simulink model "self_triggered_mpc_simulation"  (R2023a)
settings: Solver=VariableStepAuto  StartTime=0.0  StopTime=1  RelTol=1e-3
values from neighbouring files (symbols this model uses):
  param = param_setup()    [cost_cal.m]    (also in main.m; param.mat = ; self_triggered_mpc_heemels.m)
(part 2 of 2)

== stateflow chart self_triggered_mpc_simulation/Chart ==
  state self_triggered_mpc_autometica_ver
    state triggering_confirm
    state implement_mpc
      entry:
      [nTM,input]=autometica_mpc(rtm, state)
      control = input;
      during:
      [nTM,input]=autometica_mpc(rtm, state)
      control = input;
    state holding
      entry:
      control = input;
      nTM = 0;
      %holding시 nTM은 안쓰므로
      %쓰래기값을 주어도 됨
      during:
      control = input;
      nTM = 0;
    (default) -> triggering_confirm
    triggering_confirm -> implement_mpc [order 1] : [triggering == 1]
    triggering_confirm -> holding [order 2] : [triggering == 0]
    holding -> implement_mpc : [triggering == 1]
    implement_mpc -> holding : [triggering == 0]
  (default) -> self_triggered_mpc_autometica_ver
  data: TM function_input; state function_input; nTM function_output; input function_output; tm function_input; tmarr function_output; marker function_output; tm function_input; tmarr function_output; marker function_output; tm function_input; tmarr function_output; marker function_output; tm function_input; tmarr function_output; marker function_output; tm function_input; tmarr function_output; marker function_output; tm function_input; tmarr function_output; marker function_output; tm function_input; tmarr function_output; marker function_output; tm function_input; tmarr function_output; marker function_output; tm function_input; tmarr function_output; marker function_output; trigger input; rtm input; state input; nTM output; control output; input local
  function [nTM, input] = autometica_mpc(TM, state):
    | function [nTM, input] = autometica_mpc(TM, state)
    | 
    |     coder.extrinsic("optimconstr", "optimproblem", "optimvar");
    | %==========================================================================
    |  %parameter setting
    |     param = load("param.mat");
    |     param = param.param;
    |     Nl = size(TM);
    |     param.N = Nl(2);
    | %==========================================================================
    |     %implement autometica vesion
    |     prob = optimproblem;
    |     x0 = optimvar('x0', param.nx);
    |     x = optimvar('x', param.nx, param.N);
    |     u0 = optimvar('u0', param.nu);
    |     u = optimvar('u',param.nu, (param.N)-1);
    |     size(u)
    |     cost_function =x0'*param.Q*x0+u0*param.R*u0;
    |     for i=1:param.N-1
    |         cost_function = cost_function + x(:,i)'*param.Q*x(:,i) + u(:,i)'*param.R*u(:,i); % terminal cost 설정해야 됨
    |     end
    |     prob.Objective = cost_function;
    |     
    | %==========================================================================
    | % model constraints
    | 
    |     model_constr = optimconstr(param.nx,(param.N)+1);
    |     model_constr(:,1) = x(:,1) == param.A*x0 + param.B*u0;
    |     for i=1:param.N-1
    |         model_constr(:,i+1) = x(:,i+1) == param.A*x(:,i) + param.B*u(:,i);
    |     end
    |     model_constr(:,(param.N)+1) = x0 == state;
    |     prob.Constraints.model_constr = model_constr;
    |     
    | %==========================================================================
    | %terminal set constraints
    |     constT = optimconstr(30,param.autometica_Tset+1);
    |        
    |     LL = param.tildeF - param.tildeG*param.tildeK;
    |     for i= 1:param.autometica_Tset
    |         constT(:,i) = LL*(param.A_BK^(i))*param.phi(:,1:2)*x(:,param.N)<=ones(30,1);
    |     end
    |     constT(1:param.NumOfConstr,param.autometica_Tset+1) = (param.F-param.G*param.K)*x(:,param.N)<=1;
    |     prob.Constraints.ConstT = constT;
    | %==========================================================================
    | % triggering constraints
    |     SizeOfTM = size(TM);
    |     tm = TM(2:SizeOfTM(2));
    |     SizeOftm = size(tm);
    |     tmcomp = find(tm);
    |     SizeOfTmcomp = size(tmcomp);
    |     % triggering_constr = optimconstr(param.N);
    |     % triggering_constr(1) = u0 == u(:,1);
    |     % for i = 1:param.N-2
    |     %     triggering_constr(i+1) = u(:,i)==u(:,i+1); %% i+1에서 triggering하면 u(:,i)~=u(:,i+1)
    |     % end
    |     % for i = 1:SizeOfTmcomp %% required triggering time moment setting
    |     %     if tmcomp(i)==1
    |     %         triggering_constr(tmcopm(i)) = u0 ~= u(:,1);
    |     %     else
    |     %         triggering_constr(tmcomp(i)) =  u(:,tmcomp(i)-1) ~= u(:,tmcomp(i));
    |     %     end
    |     % end
    |     nontm = find(~tm); 
    |     SizeOfnontm = size(nontm);
    | %==========================================================================
    | % required trigger time moment sequence에서 triggering time moment 추가하기
    | % 이부분에서 tmarr marker를 결과로 얻는데 tmarr는 triggering time moment sequence에서
    | % triggering time moment를 추가하여 얻을 수 있는 모든 sequence를 묶어 tmarr로 받는다
    | 
    |     tmarr = [];
    |     switch SizeOfnontm(2)
    |         case 9
    |             [tmarr, marker] = trigger_plus_9(tm);
    |         case 8
    |             [tmarr, marker] = trigger_plus_8(tm);
    |         case 7
    |             [tmarr, marker] = trigger_plus_7(tm);
    |         case 6
    |             [tmarr, marker] = trigger_plus_6(tm);
    |         case 5
    |             [tmarr, marker] = trigger_plus_5(tm);
    |         case 4
    |             [tmarr, marker] = trigger_plus_4(tm);
    |         case 3
    |             [tmarr, marker] = trigger_plus_3(tm);
    |         case 2
    |             [tmarr, marker] = trigger_plus_2(tm);
    |         case 1
    |             [tmarr, marker] = trigger_plus_1(tm);
    |         case 0
    |             [tmarr, marker] = trigger_plus_0(tm);
    |     end
    | 
    | %==========================================================================
    | 
    |     SizeOftmarr = size(tmarr);
    |     SizeOfmarker = size(marker);
    | 
    |     % triggering_constr = optimconstr(param.nu, SizeOftm(2));
    |     % triggering_constr(:,1) = u0 == u(:,1); %SizeOfTM == param.N
    |     % for i = 2:SizeOftm(2)
    |     %     triggering_constr(:,i) = u(:,i-1)==u(:,i); %% i+1에서 triggering하면 u(:,i)~=u(:,i+1)
    |     % end
    |     solArr = [];
    |     fvalArr = [];
    |     exitflagArr = [];
    |     for i = 1:SizeOfmarker(2)
    |         for j = marker(i):marker(i+1)-1 
    | 
    |             tm_setting = tmarr(j,:)
    |             triggering_constr = optimconstr(param.nu, SizeOftm(2));%tm이 정해짐
    | 
    |             for k = 1:SizeOftm(2) %% required triggering time moment setting
    |                 k
    |                 if  tm_setting(k) == 0
    |                     if k ==1
    |                         triggering_constr(:,k) = u0 == u(:,1) %%optimconstr에서 ~=가 지원되지 않음
    |                         show(triggering_constr(:,k))
    |                     else
    |                         size(triggering_constr(:,k))
    |                         size(u)
    |                         triggering_constr(:,k) =  u(:,k-1) == u(:,k)
    |                         show(triggering_constr(:,i))
    |                     end
    |                 end
    |             end
    |             prob.Constraints.triggering_constr = triggering_constr
    |             [sol,fval,exitflag,output,lambda] = solve(prob)
    |             solArr = [solArr sol]
    |             fvalArr = [fvalArr fval]
    |             exitflagArr = [exitflagArr exitflag]
    |         end
    | 
    |         if ~isempty(exitflagArr==1)
    |             temp = min(fvalArr);
    |             [row, col] = find(fvalArr == temp);
    |             input=solArr(row, col).u0;
    |             nTM = tmarr(marker(i)+col-1,:);
    |             return;
    |         end
    |     end
    | 
    | end
    |     
    | 
    |     % prob.Constraints.triggering_constr = triggering_constr;
    |     % [sol,fval,exitflag,output,lambda] = solve(prob);
    |     % if exitflag == 1
    |     %     u = sol;
    |     %     t = tmcomp(1);
    |     %     nTM = tm(tmcomp(1)+1:SizeOftm)
    | % fevalArr = [];
    | %             
    | %             for c = 0:SizeOfnontmcomp %% 트리거 어디다 놓을지
    | %                 plustime = a
    | %                 while(1)
    | %                     tm(nontmcomp(c)) = 1;
    |                     
    | %                 for i = 1:SizeOfTmcomp %% required triggering time moment setting
    | %                     if tmcomp(i)==1
    | %                         triggering_constr(tmcopm(i)) = u0 ~= u(:,1);
    | %                     else
    | %                         triggering_constr(tmcomp(i)) =  u(:,tmcomp(i)-1) ~= u(:,tmcomp(i));
    | %                     end
    | %                 end
    | %                 [sol, fval, exitflag, output, lambda] = solve(prob);
    |                
    | %                 fevalArr = [feasible exitflag];
    | %                 fvalArr = [fvalArr, fval];
    | %                 solArr = [solArr, sol];
    | %             end
    | %             feasible = find(fevalArr,1);
    | %             if isempty(feasible) == 0
    | %                [row col]= min(fvalArr);
    | %                utemp = solarr(col);
    | %                u = utemp.u0;
    | %                ttemp =
  function [tmarr, marker] = trigger_plus_1(tm):
    | function [tmarr, marker] = trigger_plus_1(tm)
    |     nontm = find(~tm);
    |     SizeOfnontm = size(nontm);
    |     marker = [];
    | %--------------------------------------------------------------------------
    | % tirriger time moment +0
    |     result = [tm];
    |     temp = size(result);
    |     marker = [marker, temp(1)];
    | %--------------------------------------------------------------------------
    | % tirriger time moment +1
    |     for a1 = 1:SizeOfnontm(2)
    |         tm = result(1,:);
    |         tm(nontm(a1)) = 1;
    |         result = [result; tm];
    |         if a1 ==1
    |             temp = size(result);
    |             marker = [marker, temp(1)];
    |         end
    |     end
    |     tmarr = result;
    | end
  function [tmarr, marker] = trigger_plus_2(tm):
    | function [tmarr, marker] = trigger_plus_2(tm)
    |     nontm = find(~tm);
    |     SizeOfnontm = size(nontm);
    |     marker = [];
    | %--------------------------------------------------------------------------
    | % tirriger time moment +0
    |     result = [tm];
    |     temp = size(result);
    |     marker = [marker, temp(1)];
    | %--------------------------------------------------------------------------
    | % tirriger time moment +1
    |     for a1 = 1:SizeOfnontm(2)
    |         tm = result(1,:);
    |         tm(nontm(a1)) = 1;
    |         result = [result; tm];
    |         if a1 ==1
    |             temp = size(result);
    |             marker = [marker, temp(1)];
    |         end
    |     end
    | %--------------------------------------------------------------------------
    | % tirriger time moment +2
    |     for a1 = 1:SizeOfnontm(2)
    |         for a2 = a1+1:SizeOfnontm(2)
    |             tm = result(1,:);
    |             tm(nontm(a1)) = 1;
    |             tm(nontm(a2)) = 1;
    |             result = [result; tm];
    |             if a2 == a1+1
    |                 temp = size(result);
    |                 marker = [marker, temp(1)];
    |             end
    |         end
    |     end
    |     tmarr = result;
    | end
  function [tmarr, marker] = trigger_plus_3(tm):
    | function [tmarr, marker] = trigger_plus_3(tm)
    |     nontm = find(~tm);
    |     SizeOfnontm = size(nontm);
    |     marker = [];
    | %--------------------------------------------------------------------------
    | % tirriger time moment +0
    |     result = [tm];
    |     temp = size(result);
    |     marker = [marker, temp(1)];
    | %--------------------------------------------------------------------------
    | % tirriger time moment +1
    |     for a1 = 1:SizeOfnontm(2)
    |         tm = result(1,:);
    |         tm(nontm(a1)) = 1;
    |         result = [result; tm];
    |         if a1 ==1
    |             temp = size(result);
    |             marker = [marker, temp(1)];
    |         end
    |     end
    | %--------------------------------------------------------------------------
    | % tirriger time moment +2
    |     for a1 = 1:SizeOfnontm(2)
    |         for a2 = a1+1:SizeOfnontm(2)
    |             tm = result(1,:);
    |             tm(nontm(a1)) = 1;
    |             tm(nontm(a2)) = 1;
    |             result = [result; tm];
    |             if a2 == a1+1
    |                 temp = size(result);
    |                 marker = [marker, temp(1)];
    |             end
    |         end
    |     end
    | %--------------------------------------------------------------------------
    | % tirriger time moment +3
    | 
    |     for a1 = 1:SizeOfnontm(2)
    |         for a2 = a1+1:SizeOfnontm(2)
    |             for a3 = a2+1:SizeOfnontm(2)
    |                 tm = result(1,:);
    |                 tm(nontm(a1)) = 1;
    |                 tm(nontm(a2)) = 1;
    |                 tm(nontm(a3)) = 1;
    |                 result = [result; tm];
    |                 if a3 == a2+1
    |                     temp = size(result);
    |                     marker = [marker, temp(1)];
    |                 end
    |             end
    |         end
    |     end
    |     tmarr = result;
    | end
  function [tmarr, marker] = trigger_plus_4(tm):
    | function [tmarr, marker] = trigger_plus_4(tm)
    |     nontm = find(~tm);
    |     SizeOfnontm = size(nontm);
    |     marker = [];
    | %--------------------------------------------------------------------------
    | % tirriger time moment +0
    |     result = [tm];
    |     temp = size(result);
    |     marker = [marker, temp(1)];
    | %--------------------------------------------------------------------------
    | % tirriger time moment +1
    |     for a1 = 1:SizeOfnontm(2)
    |         tm = result(1,:);
    |         tm(nontm(a1)) = 1;
    |         result = [result; tm];
    |         if a1 ==1
    |             temp = size(result);
    |             marker = [marker, temp(1)];
    |         end
    |     end
    | %--------------------------------------------------------------------------
    | % tirriger time moment +2
    |     for a1 = 1:SizeOfnontm(2)
    |         for a2 = a1+1:SizeOfnontm(2)
    |             tm = result(1,:);
    |             tm(nontm(a1)) = 1;
    |             tm(nontm(a2)) = 1;
    |             result = [result; tm];
    |             if a2 == a1+1
    |                 temp = size(result);
    |                 marker = [marker, temp(1)];
    |             end
    |         end
    |     end
    | %--------------------------------------------------------------------------
    | % tirriger time moment +3
    | 
    |     for a1 = 1:SizeOfnontm(2)
    |         for a2 = a1+1:SizeOfnontm(2)
    |             for a3 = a2+1:SizeOfnontm(2)
    |                 tm = result(1,:);
    |                 tm(nontm(a1)) = 1;
    |                 tm(nontm(a2)) = 1;
    |                 tm(nontm(a3)) = 1;
    |                 result = [result; tm];
    |                 if a3 == a2+1
    |                     temp = size(result);
    |                     marker = [marker, temp(1)];
    |                 end
    |             end
    |         end
    |     end
    | %--------------------------------------------------------------------------
    | % tirriger time moment +4
    | 
    |     for a1 = 1:SizeOfnontm(2)
    |         for a2 = a1+1:SizeOfnontm(2)
    |             for a3 = a2+1:SizeOfnontm(2)
    |                 for a4 = a3+1:SizeOfnontm(2)
    |                     tm = result(1,:);
    |                     tm(nontm(a1)) = 1;
    |                     tm(nontm(a2)) = 1;
    |                     tm(nontm(a3)) = 1;
    |                     tm(nontm(a4)) = 1;
    |                     result = [result; tm];
    |                     if a4 == a3+1
    |                         temp = size(result);
    |                         marker = [marker, temp(1)];
    |                     end
    |                 end
    |             end
    |         end
    |     end
    |     tmarr = result;
    | end
  function [tmarr, marker] = trigger_plus_5(tm):
    | function [tmarr, marker] = trigger_plus_5(tm)
    |     nontm = find(~tm);
    |     SizeOfnontm = size(nontm);
    |     marker = [];
    | %--------------------------------------------------------------------------
    | % tirriger time moment +0
    |     result = [tm];
    |     temp = size(result);
    |     marker = [marker, temp(1)];
    | %--------------------------------------------------------------------------
    | % tirriger time moment +1
    |     for a1 = 1:SizeOfnontm(2)
    |         tm = result(1,:);
    |         tm(nontm(a1)) = 1;
    |         result = [result; tm];
    |         if a1 ==1
    |             temp = size(result);
    |             marker = [marker, temp(1)];
    |         end
    |     end
    | %--------------------------------------------------------------------------
    | % tirriger time moment +2
    |     for a1 = 1:SizeOfnontm(2)
    |         for a2 = a1+1:SizeOfnontm(2)
    |             tm = result(1,:);
    |             tm(nontm(a1)) = 1;
    |             tm(nontm(a2)) = 1;
    |             result = [result; tm];
    |             if a2 == a1+1
    |                 temp = size(result);
    |                 marker = [marker, temp(1)];
    |             end
    |         end
    |     end
    | %--------------------------------------------------------------------------
    | % tirriger time moment +3
    | 
    |     for a1 = 1:SizeOfnontm(2)
    |         for a2 = a1+1:SizeOfnontm(2)
    |             for a3 = a2+1:SizeOfnontm(2)
    |                 tm = result(1,:);
    |                 tm(nontm(a1)) = 1;
    |                 tm(nontm(a2)) = 1;
    |                 tm(nontm(a3)) = 1;
    |                 result = [result; tm];
    |                 if a3 == a2+1
    |                     temp = size(result);
    |                     marker = [marker, temp(1)];
    |                 end
    |             end
    |         end
    |     end
    | %--------------------------------------------------------------------------
    | % tirriger time moment +4
    | 
    |     for a1 = 1:SizeOfnontm(2)
    |         for a2 = a1+1:SizeOfnontm(2)
    |             for a3 = a2+1:SizeOfnontm(2)
    |                 for a4 = a3+1:SizeOfnontm(2)
    |                     tm = result(1,:);
    |                     tm(nontm(a1)) = 1;
    |                     tm(nontm(a2)) = 1;
    |                     tm(nontm(a3)) = 1;
    |                     tm(nontm(a4)) = 1;
    |                     result = [result; tm];
    |                     if a4 == a3+1
    |                         temp = size(result);
    |                         marker = [marker, temp(1)];
    |                     end
    |                 end
    |             end
    |         end
    |     end
    | %--------------------------------------------------------------------------
    | % tirriger time moment +5
    | 
    |     for a1 = 1:SizeOfnontm(2)
    |         for a2 = a1+1:SizeOfnontm(2)
    |             for a3 = a2+1:SizeOfnontm(2)
    |                 for a4 = a3+1:SizeOfnontm(2)
    |                     for a5 = a4+1:SizeOfnontm(2)
    |                         tm = result(1,:);
    |                         tm(nontm(a1)) = 1;
    |                         tm(nontm(a2)) = 1;
    |                         tm(nontm(a3)) = 1;
    |                         tm(nontm(a4)) = 1;
    |                         tm(nontm(a5)) = 1;
    |                         result = [result; tm];
    |                         if a5 == a4+1
    |                             temp = size(result);
    |                             marker = [marker, temp(1)];
    |                         end
    |                     end
    |                 end
    |             end
    |         end
    |     end
    |     tmarr = result;
    | end
  function [tmarr, marker] = trigger_plus_6(tm):
    | function [tmarr, marker] = trigger_plus_6(tm)
    |     nontm = find(~tm);
    |     SizeOfnontm = size(nontm);
    |     marker = [];
    | %--------------------------------------------------------------------------
    | % tirriger time moment +0
    |     result = [tm];
    |     temp = size(result);
    |     marker = [marker, temp(1)];
    | %--------------------------------------------------------------------------
    | % tirriger time moment +1
    |     for a1 = 1:SizeOfnontm(2)
    |         tm = result(1,:);
    |         tm(nontm(a1)) = 1;
    |         result = [result; tm];
    |         if a1 ==1
    |             temp = size(result);
    |             marker = [marker, temp(1)];
    |         end
    |     end
    | %--------------------------------------------------------------------------
    | % tirriger time moment +2
    |     for a1 = 1:SizeOfnontm(2)
    |         for a2 = a1+1:SizeOfnontm(2)
    |             tm = result(1,:);
    |             tm(nontm(a1)) = 1;
    |             tm(nontm(a2)) = 1;
    |             result = [result; tm];
    |             if a2 == a1+1
    |                 temp = size(result);
    |                 marker = [marker, temp(1)];
    |             end
    |         end
    |     end
    | %--------------------------------------------------------------------------
    | % tirriger time moment +3
    | 
    |     for a1 = 1:SizeOfnontm(2)
    |         for a2 = a1+1:SizeOfnontm(2)
    |             for a3 = a2+1:SizeOfnontm(2)
    |                 tm = result(1,:);
    |                 tm(nontm(a1)) = 1;
    |                 tm(nontm(a2)) = 1;
    |                 tm(nontm(a3)) = 1;
    |                 result = [result; tm];
    |                 if a3 == a2+1
    |                     temp = size(result);
    |                     marker = [marker, temp(1)];
    |                 end
    |             end
    |         end
    |     end
    | %--------------------------------------------------------------------------
    | % tirriger time moment +4
    | 
    |     for a1 = 1:SizeOfnontm(2)
    |         for a2 = a1+1:SizeOfnontm(2)
    |             for a3 = a2+1:SizeOfnontm(2)
    |                 for a4 = a3+1:SizeOfnontm(2)
    |                     tm = result(1,:);
    |                     tm(nontm(a1)) = 1;
    |                     tm(nontm(a2)) = 1;
    |                     tm(nontm(a3)) = 1;
    |                     tm(nontm(a4)) = 1;
    |                     result = [result; tm];
    |                     if a4 == a3+1
    |                         temp = size(result);
    |                         marker = [marker, temp(1)];
    |                     end
    |                 end
    |             end
    |         end
    |     end
    | %--------------------------------------------------------------------------
    | % tirriger time moment +5
    | 
    |     for a1 = 1:SizeOfnontm(2)
    |         for a2 = a1+1:SizeOfnontm(2)
    |             for a3 = a2+1:SizeOfnontm(2)
    |                 for a4 = a3+1:SizeOfnontm(2)
    |                     for a5 = a4+1:SizeOfnontm(2)
    |                         tm = result(1,:);
    |                         tm(nontm(a1)) = 1;
    |                         tm(nontm(a2)) = 1;
    |                         tm(nontm(a3)) = 1;
    |                         tm(nontm(a4)) = 1;
    |                         tm(nontm(a5)) = 1;
    |                         result = [result; tm];
    |                         if a5 == a4+1
    |                             temp = size(result);
    |                             marker = [marker, temp(1)];
    |                         end
    |                     end
    |                 end
    |             end
    |         end
    |     end
    | %--------------------------------------------------------------------------
    | % tirriger time moment +6
    | 
    |     for a1 = 1:SizeOfnontm(2)
    |         for a2 = a1+1:SizeOfnontm(2)
    |             for a3 = a2+1:SizeOfnontm(2)
    |                 for a4 = a3+1:SizeOfnontm(2)
    |                     for a5 = a4+1:SizeOfnontm(2)
    |                         for a6 = a5+1:SizeOfnontm(2)
    |                             tm = result(1,:);
    |                             tm(nontm(a1)) = 1;
    |                             tm(nontm(a2)) = 1;
    |                             tm(nontm(a3)) = 1;
    |                             tm(nontm(a4)) = 1;
    |                             tm(nontm(a5)) = 1;
    |                             tm(nontm(a6)) = 1;
    |                             result = [result; tm];
    |                             if a6 == a5+1
    |                                 temp = size(result);
    |                                 marker = [marker, temp(1)];
    |                             end
    |                         end
    |                     end
    |                 end
    |             end
    |         end
    |     end
    |     tmarr = result;
    | end
  function [tmarr, marker] = trigger_plus_7(tm):
    | function [tmarr, marker] = trigger_plus_7(tm)
    |     nontm = find(~tm);
    |     SizeOfnontm = size(nontm);
    |     marker = [];
    | %--------------------------------------------------------------------------
    | % tirriger time moment +0
    |     result = [tm];
    |     temp = size(result);
    |     marker = [marker, temp(1)];
    | %--------------------------------------------------------------------------
    | % tirriger time moment +1
    |     for a1 = 1:SizeOfnontm(2)
    |         tm = result(1,:);
    |         tm(nontm(a1)) = 1;
    |         result = [result; tm];
    |         if a1 ==1
    |             temp = size(result);
    |             marker = [marker, temp(1)];
    |         end
    |     end
    | %--------------------------------------------------------------------------
    | % tirriger time moment +2
    |     for a1 = 1:SizeOfnontm(2)
    |         for a2 = a1+1:SizeOfnontm(2)
    |             tm = result(1,:);
    |             tm(nontm(a1)) = 1;
    |             tm(nontm(a2)) = 1;
    |             result = [result; tm];
    |             if a2 == a1+1
    |                 temp = size(result);
    |                 marker = [marker, temp(1)];
    |             end
    |         end
    |     end
    | %--------------------------------------------------------------------------
    | % tirriger time moment +3
    | 
    |     for a1 = 1:SizeOfnontm(2)
    |         for a2 = a1+1:SizeOfnontm(2)
    |             for a3 = a2+1:SizeOfnontm(2)
    |                 tm = result(1,:);
    |                 tm(nontm(a1)) = 1;
    |                 tm(nontm(a2)) = 1;
    |                 tm(nontm(a3)) = 1;
    |                 result = [result; tm];
    |                 if a3 == a2+1
    |                     temp = size(result);
    |                     marker = [marker, temp(1)];
    |                 end
    |             end
    |         end
    |     end
    | %--------------------------------------------------------------------------
    | % tirriger time moment +4
    | 
    |     for a1 = 1:SizeOfnontm(2)
    |         for a2 = a1+1:SizeOfnontm(2)
    |             for a3 = a2+1:SizeOfnontm(2)
    |                 for a4 = a3+1:SizeOfnontm(2)
    |                     tm = result(1,:);
    |                     tm(nontm(a1)) = 1;
    |                     tm(nontm(a2)) = 1;
    |                     tm(nontm(a3)) = 1;
    |                     tm(nontm(a4)) = 1;
    |                     result = [result; tm];
    |                     if a4 == a3+1
    |                         temp = size(result);
    |                         marker = [marker, temp(1)];
    |                     end
    |                 end
    |             end
    |         end
    |     end
    | %--------------------------------------------------------------------------
    | % tirriger time moment +5
    | 
    |     for a1 = 1:SizeOfnontm(2)
    |         for a2 = a1+1:SizeOfnontm(2)
    |             for a3 = a2+1:SizeOfnontm(2)
    |                 for a4 = a3+1:SizeOfnontm(2)
    |                     for a5 = a4+1:SizeOfnontm(2)
    |                         tm = result(1,:);
    |                         tm(nontm(a1)) = 1;
    |                         tm(nontm(a2)) = 1;
    |                         tm(nontm(a3)) = 1;
    |                         tm(nontm(a4)) = 1;
    |                         tm(nontm(a5)) = 1;
    |                         result = [result; tm];
    |                         if a5 == a4+1
    |                             temp = size(result);
    |                             marker = [marker, temp(1)];
    |                         end
    |                     end
    |                 end
    |             end
    |         end
    |     end
    | %--------------------------------------------------------------------------
    | % tirriger time moment +6
    | 
    |     for a1 = 1:SizeOfnontm(2)
    |         for a2 = a1+1:SizeOfnontm(2)
    |             for a3 = a2+1:SizeOfnontm(2)
    |                 for a4 = a3+1:SizeOfnontm(2)
    |                     for a5 = a4+1:SizeOfnontm(2)
    |                         for a6 = a5+1:SizeOfnontm(2)
    |                             tm = result(1,:);
    |                             tm(nontm(a1)) = 1;
    |                             tm(nontm(a2)) = 1;
    |                             tm(nontm(a3)) = 1;
    |                             tm(nontm(a4)) = 1;
    |                             tm(nontm(a5)) = 1;
    |                             tm(nontm(a6)) = 1;
    |                             result = [result; tm];
    |                             if a6 == a5+1
    |                                 temp = size(result);
    |                                 marker = [marker, temp(1)];
    |                             end
    |                         end
    |                     end
    |                 end
    |             end
    |         end
    |     end
    | %--------------------------------------------------------------------------
    | % tirriger time moment +7
    | 
    |     for a1 = 1:SizeOfnontm(2)
    |         for a2 = a1+1:SizeOfnontm(2)
    |             for a3 = a2+1:SizeOfnontm(2)
    |                 for a4 = a3+1:SizeOfnontm(2)
    |                     for a5 = a4+1:SizeOfnontm(2)
    |                         for a6 = a5+1:SizeOfnontm(2)
    |                             for a7 = a6+1:SizeOfnontm(2)
    |                                 tm = result(1,:);
    |                                 tm(nontm(a1)) = 1;
    |                                 tm(nontm(a2)) = 1;
    |                                 tm(nontm(a3)) = 1;
    |                                 tm(nontm(a4)) = 1;
    |                                 tm(nontm(a5)) = 1;
    |                                 tm(nontm(a6)) = 1;
    |                                 tm(nontm(a7)) = 1;
    |                                 result = [result; tm];
    |                                 if a7 == a6+1
    |                                     temp = size(result);
    |                                     marker = [marker, temp(1)];
    |                                 end
    |                             end
    |                         end
    |                     end
    |                 end
    |             end
    |         end
    |     end
    |     tmarr = result;
    | end
  function [tmarr, marker] = trigger_plus_8(tm):
    | function [tmarr, marker] = trigger_plus_8(tm)
    |     nontm = find(~tm);
    |     SizeOfnontm = size(nontm);
    |     marker = [];
    | %--------------------------------------------------------------------------
    | % tirriger time moment +0
    |     result = [tm];
    |     temp = size(result);
    |     marker = [marker, temp(1)];
    | %--------------------------------------------------------------------------
    | % tirriger time moment +1
    |     for a1 = 1:SizeOfnontm(2)
    |         tm = result(1,:);
    |         tm(nontm(a1)) = 1;
    |         result = [result; tm];
    |         if a1 ==1
    |             temp = size(result);
    |             marker = [marker, temp(1)];
    |         end
    |     end
    | %--------------------------------------------------------------------------
    | % tirriger time moment +2
    |     for a1 = 1:SizeOfnontm(2)
    |         for a2 = a1+1:SizeOfnontm(2)
    |             tm = result(1,:);
    |             tm(nontm(a1)) = 1;
    |             tm(nontm(a2)) = 1;
    |             result = [result; tm];
    |             if a2 == a1+1
    |                 temp = size(result);
    |                 marker = [marker, temp(1)];
    |             end
    |         end
    |     end
    | %--------------------------------------------------------------------------
    | % tirriger time moment +3
    | 
    |     for a1 = 1:SizeOfnontm(2)
    |         for a2 = a1+1:SizeOfnontm(2)
    |             for a3 = a2+1:SizeOfnontm(2)
    |                 tm = result(1,:);
    |                 tm(nontm(a1)) = 1;
    |                 tm(nontm(a2)) = 1;
    |                 tm(nontm(a3)) = 1;
    |                 result = [result; tm];
    |                 if a3 == a2+1
    |                     temp = size(result);
    |                     marker = [marker, temp(1)];
    |                 end
    |             end
    |         end
    |     end
    | %--------------------------------------------------------------------------
    | % tirriger time moment +4
    | 
    |     for a1 = 1:SizeOfnontm(2)
    |         for a2 = a1+1:SizeOfnontm(2)
    |             for a3 = a2+1:SizeOfnontm(2)
    |                 for a4 = a3+1:SizeOfnontm(2)
    |                     tm = result(1,:);
    |                     tm(nontm(a1)) = 1;
    |                     tm(nontm(a2)) = 1;
    |                     tm(nontm(a3)) = 1;
    |                     tm(nontm(a4)) = 1;
    |                     result = [result; tm];
    |                     if a4 == a3+1
    |                         temp = size(result);
    |                         marker = [marker, temp(1)];
    |                     end
    |                 end
    |             end
    |         end
    |     end
    | %--------------------------------------------------------------------------
    | % tirriger time moment +5
    | 
    |     for a1 = 1:SizeOfnontm(2)
    |         for a2 = a1+1:SizeOfnontm(2)
    |             for a3 = a2+1:SizeOfnontm(2)
    |                 for a4 = a3+1:SizeOfnontm(2)
    |                     for a5 = a4+1:SizeOfnontm(2)
    |                         tm = result(1,:);
    |                         tm(nontm(a1)) = 1;
    |                         tm(nontm(a2)) = 1;
    |                         tm(nontm(a3)) = 1;
    |                         tm(nontm(a4)) = 1;
    |                         tm(nontm(a5)) = 1;
    |                         result = [result; tm];
    |                         if a5 == a4+1
    |                             temp = size(result);
    |                             marker = [marker, temp(1)];
    |                         end
    |                     end
    |                 end
    |             end
    |         end
    |     end
    | %--------------------------------------------------------------------------
    | % tirriger time moment +6
    | 
    |     for a1 = 1:SizeOfnontm(2)
    |         for a2 = a1+1:SizeOfnontm(2)
    |             for a3 = a2+1:SizeOfnontm(2)
    |                 for a4 = a3+1:SizeOfnontm(2)
    |                     for a5 = a4+1:SizeOfnontm(2)
    |                         for a6 = a5+1:SizeOfnontm(2)
    |                             tm = result(1,:);
    |                             tm(nontm(a1)) = 1;
    |                             tm(nontm(a2)) = 1;
    |                             tm(nontm(a3)) = 1;
    |                             tm(nontm(a4)) = 1;
    |                             tm(nontm(a5)) = 1;
    |                             tm(nontm(a6)) = 1;
    |                             result = [result; tm];
    |                             if a6 == a5+1
    |                                 temp = size(result);
    |                                 marker = [marker, temp(1)];
    |                             end
    |                         end
    |                     end
    |                 end
    |             end
    |         end
    |     end
    | %--------------------------------------------------------------------------
    | % tirriger time moment +7
    | 
    |     for a1 = 1:SizeOfnontm(2)
    |         for a2 = a1+1:SizeOfnontm(2)
    |             for a3 = a2+1:SizeOfnontm(2)
    |                 for a4 = a3+1:SizeOfnontm(2)
    |                     for a5 = a4+1:SizeOfnontm(2)
    |                         for a6 = a5+1:SizeOfnontm(2)
    |                             for a7 = a6+1:SizeOfnontm(2)
    |                                 tm = result(1,:);
    |                                 tm(nontm(a1)) = 1;
    |                                 tm(nontm(a2)) = 1;
    |                                 tm(nontm(a3)) = 1;
    |                                 tm(nontm(a4)) = 1;
    |                                 tm(nontm(a5)) = 1;
    |                                 tm(nontm(a6)) = 1;
    |                                 tm(nontm(a7)) = 1;
    |                                 result = [result; tm];
    |                                 if a7 == a6+1
    |                                     temp = size(result);
    |                                     marker = [marker, temp(1)];
    |                                 end
    |                             end
    |                         end
    |                     end
    |                 end
    |             end
    |         end
    |     end
    | %--------------------------------------------------------------------------
    | % tirriger time moment +8
    | 
    |     for a1 = 1:SizeOfnontm(2)
    |         for a2 = a1+1:SizeOfnontm(2)
    |             for a3 = a2+1:SizeOfnontm(2)
    |                 for a4 = a3+1:SizeOfnontm(2)
    |                     for a5 = a4+1:SizeOfnontm(2)
    |                         for a6 = a5+1:SizeOfnontm(2)
    |                             for a7 = a6+1:SizeOfnontm(2)
    |                                 for a8 = a7+1:SizeOfnontm(2)
    |                                     tm = result(1,:);
    |                                     tm(nontm(a1)) = 1;
    |                                     tm(nontm(a2)) = 1;
    |                                     tm(nontm(a3)) = 1;
    |                                     tm(nontm(a4)) = 1;
    |                                     tm(nontm(a5)) = 1;
    |                                     tm(nontm(a6)) = 1;
    |                                     tm(nontm(a7)) = 1;
    |                                     tm(nontm(a8)) = 1;
    |                                     result = [result; tm];
    |                                     if a8 == a7+1
    |                                         temp = size(result);
    |                                         marker = [marker, temp(1)];
    |                                     end
    |                                 end
    |                             end
    |                         end
    |                     end
    |                 end
    |             end
    |         end
    |     end
    |     tmarr = result;
    | end
  function [tmarr, marker] = trigger_plus_9(tm):
    | function [tmarr, marker] = trigger_plus_9(tm)
    |     nontm = find(~tm);
    |     SizeOfnontm = size(nontm);
    |     marker = [];
    | %--------------------------------------------------------------------------
    | % tirriger time moment +0
    |     result = [tm];
    |     temp = size(result);
    |     marker = [marker, temp(1)];
    | %--------------------------------------------------------------------------
    | % tirriger time moment +1
    |     for a1 = 1:SizeOfnontm(2)
    |         tm = result(1,:);
    |         tm(nontm(a1)) = 1;
    |         result = [result; tm];
    |         if a1 ==1
    |             temp = size(result);
    |             marker = [marker, temp(1)];
    |         end
    |     end
    | %--------------------------------------------------------------------------
    | % tirriger time moment +2
    |     for a1 = 1:SizeOfnontm(2)
    |         for a2 = a1+1:SizeOfnontm(2)
    |             tm = result(1,:);
    |             tm(nontm(a1)) = 1;
    |             tm(nontm(a2)) = 1;
    |             result = [result; tm];
    |             if a2 == a1+1
    |                 temp = size(result);
    |                 marker = [marker, temp(1)];
    |             end
    |         end
    |     end
    | %--------------------------------------------------------------------------
    | % tirriger time moment +3
    | 
    |     for a1 = 1:SizeOfnontm(2)
    |         for a2 = a1+1:SizeOfnontm(2)
    |             for a3 = a2+1:SizeOfnontm(2)
    |                 tm = result(1,:);
    |                 tm(nontm(a1)) = 1;
    |                 tm(nontm(a2)) = 1;
    |                 tm(nontm(a3)) = 1;
    |                 result = [result; tm];
    |                 if a3 == a2+1
    |                     temp = size(result);
    |                     marker = [marker, temp(1)];
    |                 end
    |             end
    |         end
    |     end
    | %--------------------------------------------------------------------------
    | % tirriger time moment +4
    | 
    |     for a1 = 1:SizeOfnontm(2)
    |         for a2 = a1+1:SizeOfnontm(2)
    |             for a3 = a2+1:SizeOfnontm(2)
    |                 for a4 = a3+1:SizeOfnontm(2)
    |                     tm = result(1,:);
    |                     tm(nontm(a1)) = 1;
    |                     tm(nontm(a2)) = 1;
    |                     tm(nontm(a3)) = 1;
    |                     tm(nontm(a4)) = 1;
    |                     result = [result; tm];
    |                     if a4 == a3+1
    |                         temp = size(result);
    |                         marker = [marker, temp(1)];
    |                     end
    |                 end
    |             end
    |         end
    |     end
    | %--------------------------------------------------------------------------
    | % tirriger time moment +5
    | 
    |     for a1 = 1:SizeOfnontm(2)
    |         for a2 = a1+1:SizeOfnontm(2)
    |             for a3 = a2+1:SizeOfnontm(2)
    |                 for a4 = a3+1:SizeOfnontm(2)
    |                     for a5 = a4+1:SizeOfnontm(2)
    |                         tm = result(1,:);
    |                         tm(nontm(a1)) = 1;
    |                         tm(nontm(a2)) = 1;
    |                         tm(nontm(a3)) = 1;
    |                         tm(nontm(a4)) = 1;
    |                         tm(nontm(a5)) = 1;
    |                         result = [result; tm];
    |                         if a5 == a4+1
    |                             temp = size(result);
    |                             marker = [marker, temp(1)];
    |                         end
    |                     end
    |                 end
    |             end
    |         end
    |     end
    | %--------------------------------------------------------------------------
    | % tirriger time moment +6
    | 
    |     for a1 = 1:SizeOfnontm(2)
    |         for a2 = a1+1:SizeOfnontm(2)
    |             for a3 = a2+1:SizeOfnontm(2)
    |                 for a4 = a3+1:SizeOfnontm(2)
    |                     for a5 = a4+1:SizeOfnontm(2)
    |                         for a6 = a5+1:SizeOfnontm(2)
    |                             tm = result(1,:);
    |                             tm(nontm(a1)) = 1;
    |                             tm(nontm(a2)) = 1;
    |                             tm(nontm(a3)) = 1;
    |                             tm(nontm(a4)) = 1;
    |                             tm(nontm(a5)) = 1;
    |                             tm(nontm(a6)) = 1;
    |                             result = [result; tm];
    |                             if a6 == a5+1
    |                                 temp = size(result);
    |                                 marker = [marker, temp(1)];
    |                             end
    |                         end
    |                     end
    |                 end
    |             end
    |         end
    |     end
    | %--------------------------------------------------------------------------
    | % tirriger time moment +7
    | 
    |     for a1 = 1:SizeOfnontm(2)
    |         for a2 = a1+1:SizeOfnontm(2)
    |             for a3 = a2+1:SizeOfnontm(2)
    |                 for a4 = a3+1:SizeOfnontm(2)
    |                     for a5 = a4+1:SizeOfnontm(2)
    |                         for a6 = a5+1:SizeOfnontm(2)
    |                             for a7 = a6+1:SizeOfnontm(2)
    |                                 tm = result(1,:);
    |                                 tm(nontm(a1)) = 1;
    |                                 tm(nontm(a2)) = 1;
    |                                 tm(nontm(a3)) = 1;
    |                                 tm(nontm(a4)) = 1;
    |                                 tm(nontm(a5)) = 1;
    |                                 tm(nontm(a6)) = 1;
    |                                 tm(nontm(a7)) = 1;
    |                                 result = [result; tm];
    |                                 if a7 == a6+1
    |                                     temp = size(result);
    |                                     marker = [marker, temp(1)];
    |                                 end
    |                             end
    |                         end
    |                     end
    |                 end
    |             end
    |         end
    |     end
    | %--------------------------------------------------------------------------
    | % tirriger time moment +8
    | 
    |     for a1 = 1:SizeOfnontm(2)
    |         for a2 = a1+1:SizeOfnontm(2)
    |             for a3 = a2+1:SizeOfnontm(2)
    |                 for a4 = a3+1:SizeOfnontm(2)
    |                     for a5 = a4+1:SizeOfnontm(2)
    |                         for a6 = a5+1:SizeOfnontm(2)
    |                             for a7 = a6+1:SizeOfnontm(2)
    |                                 for a8 = a7+1:SizeOfnontm(2)
    |                                     tm = result(1,:);
    |                                     tm(nontm(a1)) = 1;
    |                                     tm(nontm(a2)) = 1;
    |                                     tm(nontm(a3)) = 1;
    |                                     tm(nontm(a4)) = 1;
    |                                     tm(nontm(a5)) = 1;
    |                                     tm(nontm(a6)) = 1;
    |                                     tm(nontm(a7)) = 1;
    |                                     tm(nontm(a8)) = 1;
    |                                     result = [result; tm];
    |                                     if a8 == a7+1
    |                                         temp = size(result);
    |                                         marker = [marker, temp(1)];
    |                                     end
    |                                 end
    |                             end
    |                         end
    |                     end
    |                 end
    |             end
    |         end
    |     end
    | %--------------------------------------------------------------------------
    | % tirriger time moment +9
    | 
    |     for a1 = 1:SizeOfnontm(2)
    |         for a2 = a1+1:SizeOfnontm(2)
    |             for a3 = a2+1:SizeOfnontm(2)
    |                 for a4 = a3+1:SizeOfnontm(2)
    |                     for a5 = a4+1:SizeOfnontm(2)
    |                         for a6 = a5+1:SizeOfnontm(2)
    |                             for a7 = a6+1:SizeOfnontm(2)
    |                                 for a8 = a7+1:SizeOfnontm(2)
    |                                     for a9 = a8+1:SizeOfnontm(2)
    |                                         tm = result(1,:);
    |                                         tm(nontm(a1)) = 1;
    |                                         tm(nontm(a2)) = 1;
    |                                         tm(nontm(a3)) = 1;
    |                                         tm(nontm(a4)) = 1;
    |                                         tm(nontm(a5)) = 1;
    |                                         tm(nontm(a6)) = 1;
    |                                         tm(nontm(a7)) = 1;
    |                                         tm(nontm(a8)) = 1;
    |                                         tm(nontm(a9)) = 1;
    |                                         result = [result; tm];
    |                                         if a9 == a8+1
    |                                             temp = size(result);
    |                                             marker = [marker, temp(1)];
    |                                         end
    |                                     end
    |                                 end
    |                             end
    |                         end
    |                     end
    |                 end
    |             end
    |         end
    |     end
    |     tmarr = result;
    | endfunction trigger_plus_9
